simulink model "Examenmodelado_Campoy"  (R2023a)
settings: Solver=VariableStepAuto  StartTime=0.0  StopTime=10.0  RelTol=1e-3
libraries: fl_lib x14, nesl_utility x6, slpidlib x1
settings Model: Creator=marco  LastModifiedBy=marco

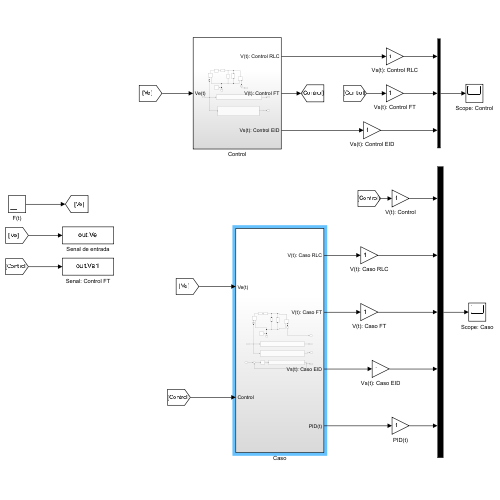
[thumbnail: Simulink's stored preview of the top-level diagram]
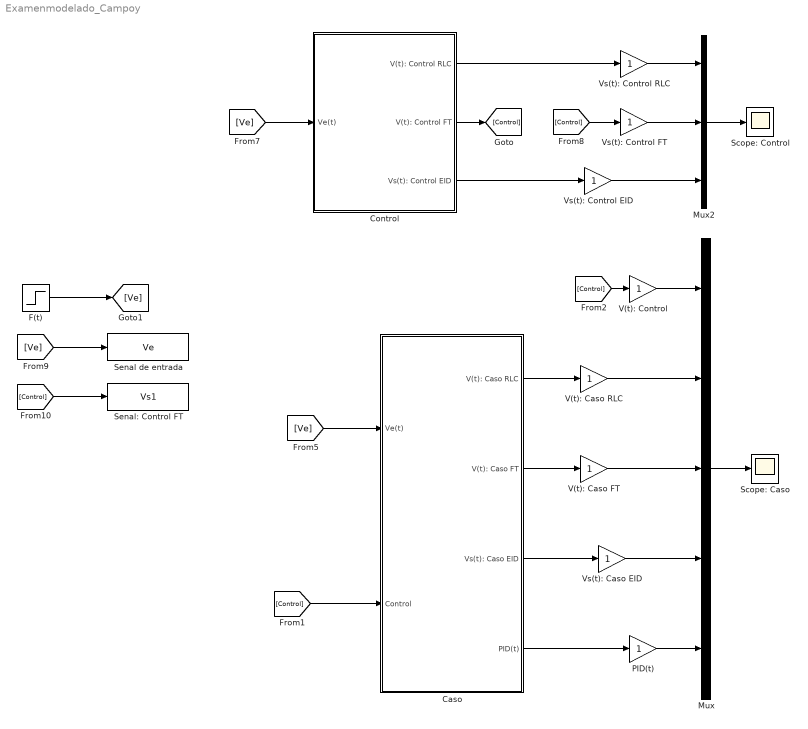
== system Examenmodelado_Campoy ==
  Caso : Subsystem
  Control : Subsystem
  F(t) : Step  SampleTime=0
  Mux : Mux  Inputs=5
  Mux2 : Mux  Inputs=3
  PID(t) : Gain
  Scope: Caso : Scope
  Scope: Control : Scope
  Senal de entrada : ToWorkspace  VariableName=Ve  SampleTime=-1
  Senal: Control FT : ToWorkspace  VariableName=Vs1  SampleTime=-1
  V(t): Caso FT : Gain
  V(t): Caso RLC : Gain
  V(t): Control : Gain
  Vs(t): Caso EID : Gain
  Vs(t): Control EID : Gain
  Vs(t): Control FT : Gain
  Vs(t): Control RLC : Gain
  wires:
  Vs(t): Control EID/1 -> Mux2/3
  V(t): Control/1 -> Mux/1
  Control/2(V(t): Control FT) -> [Control]
  Vs(t): Control RLC/1 -> Mux2/1
  Caso/3(Vs(t): Caso EID) -> Vs(t): Caso EID/1
  [Control] -> Vs(t): Control FT/1
  [Control] -> Senal: Control FT/1
  [Ve] -> Control/1(Ve(t))
  Control/1(V(t): Control RLC) -> Vs(t): Control RLC/1
  Vs(t): Control FT/1 -> Mux2/2
  Mux2/1 -> Scope: Control/1
  Control/3(Vs(t): Control EID) -> Vs(t): Control EID/1
  F(t)/1 -> [Ve]
  Mux/1 -> Scope: Caso/1
  [Ve] -> Senal de entrada/1
  [Control] -> V(t): Control/1
  Caso/2(V(t): Caso FT) -> V(t): Caso FT/1
  Caso/4(PID(t)) -> PID(t)/1
  Vs(t): Caso EID/1 -> Mux/4
  PID(t)/1 -> Mux/5
  [Control] -> Caso/2(Control)
  [Ve] -> Caso/1(Ve(t))
  Caso/1(V(t): Caso RLC) -> V(t): Caso RLC/1
  V(t): Caso RLC/1 -> Mux/2
  V(t): Caso FT/1 -> Mux/3

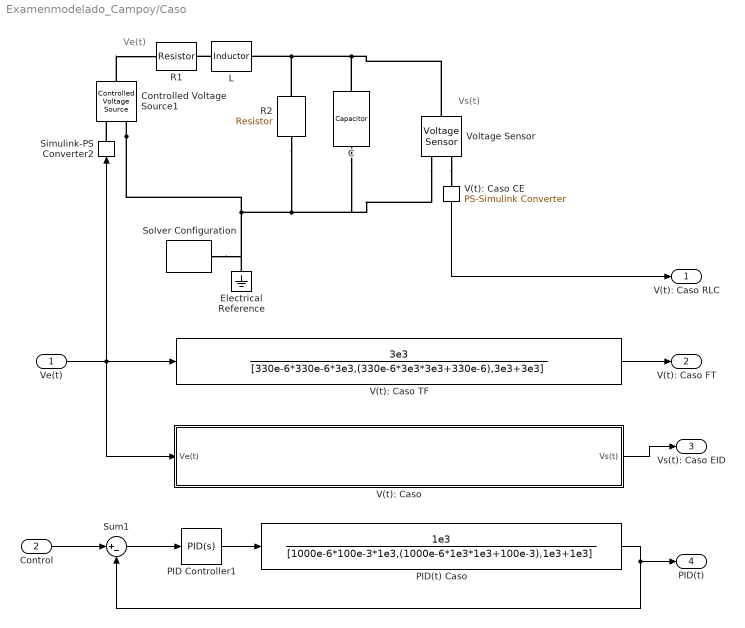
== system Examenmodelado_Campoy/Caso ==
  note: Ve(t)
  note: Vs(t)
  Ve(t) : Inport
  Control : Inport  Port=2
  C : fl_lib/Electrical/Electrical Elements/Capacitor  c=330 uF  r=1e-6 Ohm  g=0 1/Ohm  i_specify=off  i_priority=None  i=0 A  i_nominal_specify=off  i_nominal_unit=A  i_nominal_value=1  v_specify=off  v_priority=None  v=0 V  v_nominal_specify=off  v_nominal_unit=V  v_nominal_value=1  vc_specify=off  vc_priority=High  vc=0 V  vc_nominal_specify=off  vc_nominal_unit=V  vc_nominal_value=1
  Controlled Voltage Source1 : fl_lib/Electrical/Electrical Sources/Controlled Voltage Source
  Electrical Reference : fl_lib/Electrical/Electrical Elements/Electrical Reference
  L : fl_lib/Electrical/Electrical Elements/Inductor  l=330 uH  r=0 Ohm  g=1e-9 1/Ohm  i_specify=off  i_priority=None  i=0 A  i_nominal_specify=off  i_nominal_unit=A  i_nominal_value=1  v_specify=off  v_priority=None  v=0 V  v_nominal_specify=off  v_nominal_unit=V  v_nominal_value=1  i_L_specify=off  i_L_priority=High  i_L=0 A  i_L_nominal_specify=off  i_L_nominal_unit=A  i_L_nominal_value=1
  PID Controller1 : slpidlib/PID Controller  Controller=PID  Form=Parallel  TimeDomain=Continuous-time  UseExternalTs=off  SampleTime=-1  IntegratorMethod=Forward Euler  FilterMethod=Forward Euler  ControllerParametersSource=internal  P=1300.02549518255  I=307059.160027012  UseKiTs=off  D=0.293182881329496  N=7462.72432566653  UseFilter=on  TunerSelectOption=Frequency Response Based  InitialConditionSource=internal  InitialConditionForIntegrator=0  InitialConditionForFilter=0  DifferentiatorICPrevScaledInput=0  ExternalReset=none  TrackingMode=off  Kt=1  LimitOutput=off  SatLimitsSource=internal  UpperSaturationLimit=inf  LowerSaturationLimit=-inf  LinearizeAsGain=on  AntiWindupMode=none  Kb=1  LimitIntegrator=off  UpperIntegratorSaturationLimit=inf  LowerIntegratorSaturationLimit=-inf  POutMin=[]  POutMax=[]  IOutMin=[]  IOutMax=[]  DOutMin=[]  DOutMax=[]  NOutMin=[]  NOutMax=[]  SumOutMin=[]  SumOutMax=[]  SaturationOutMin=[]  SaturationOutMax=[]  PParamMin=[]  PParamMax=[]  IParamMin=[]  IParamMax=[]  DParamMin=[]  DParamMax=[]  NParamMin=[]  NParamMax=[]  KbParamMin=[]  KbParamMax=[]  KtParamMin=[]  KtParamMax=[]  KbOutMin=[]  KbOutMax=[]  KtOutMin=[]  KtOutMax=[]  IntegratorOutMin=[]  IntegratorOutMax=[]  FilterOutMin=[]  FilterOutMax=[]  SumI1OutMin=[]  SumI1OutMax=[]  SumI2OutMin=[]  SumI2OutMax=[]  SumI3OutMin=[]  SumI3OutMax=[]  SumI4OutMin=[]  SumI4OutMax=[]  SumDOutMin=[]  SumDOutMax=[]  DifferentiatorOutMin=[]  DifferentiatorOutMax=[]  FilterDiffOutCoefMin=[]  FilterDiffOutCoefMax=[]  ReciprocalOutMin=[]  ReciprocalOutMax=[]  SumDenOutMin=[]  SumDenOutMax=[]  SumNumOutMin=[]  SumNumOutMax=[]  DivideOutMin=[]  DivideOutMax=[]  UdiffTsProdOutMin=[]  UdiffTsProdOutMax=[]  NTsProdOutMin=[]  NTsProdOutMax=[]  UintegralTsProdOutMin=[]  UintegralTsProdOutMax=[]  UngainTsProdOutMin=[]  UngainTsProdOutMax=[]  ClampingZeroOutDataTypeStr=Inherit: Inherit via back propagation  ClampingZeroOutMin=[]  ClampingZeroOutMax=[]  FilterDenConstantOutDataTypeStr=Inherit: Inherit via back propagation  FilterDenConstantOutMin=[]  FilterDenConstantOutMax=[]  PCopyOutDataTypeStr=Inherit: Inherit via back propagation  PCopyOutMin=[]  PCopyOutMax=[]  NCopyOutDataTypeStr=Inherit: Inherit via back propagation  NCopyOutMin=[]  NCopyOutMax=[]  IntegratorContinuousStateAttributes=''  IntegratorStateMustResolveToSignalObject=off  IntegratorRTWStateStorageClass=Auto  FilterContinuousStateAttributes=''  FilterStateMustResolveToSignalObject=off  FilterRTWStateStorageClass=Auto  ParallelPVariant=InternalParameters  IdealPVariant=Disabled  IVariant=InternalParameters  DVariant=InternalParameters  IntegratorVariant=Continuous  SatVariant=Disabled  AWVariant=Passthrough  PCopyVariant=Disabled  TRVariant=Disabled  FdbkBlocksVariant=Forward  IdealPFdbkVariant=Disabled  SatFdbkVariant=Disabled  DerivativeFilterVariant=ContFilter  NVariant=InternalParameters  NCopyVariant=Disabled  FilterICVariant=InternalICsFilter  IntegratorICVariant=InternalICs  ExternalResetVariant=Disabled  TRSumVariant=Passthrough  SumFdbkVariant=Disabled  SumVariant=Sum_PID  TsampFilterVariant=InternalTs  TsampNgainVariant=Passthrough  TsampIntegralVariant=Disabled_SignalSpec  ExternalSaturationOutDataTypeStr=Inherit: Same as second input
  PID(t) Caso : TransferFcn  Numerator=[1e3]  Denominator=[1000e-6*100e-3*1e3,(1000e-6*1e3*1e3+100e-3),1e3+1e3]
  R1 : fl_lib/Electrical/Electrical Elements/Resistor  R=3 kOhm  i_specify=off  i_priority=None  i=0 A  i_nominal_specify=off  i_nominal_unit=A  i_nominal_value=1  v_specify=off  v_priority=None  v=0 V  v_nominal_specify=off  v_nominal_unit=V  v_nominal_value=1
  R2 : fl_lib/Electrical/Electrical Elements/Resistor  R=3 kOhm  i_specify=off  i_priority=None  i=0 A  i_nominal_specify=off  i_nominal_unit=A  i_nominal_value=1  v_specify=off  v_priority=None  v=0 V  v_nominal_specify=off  v_nominal_unit=V  v_nominal_value=1
  Simulink-PS Converter2 : nesl_utility/Simulink-PS Converter  PhysicalDomain=network_engine_domain  SubClassName=ps_input  LeftPortType=input  RightPortType=output  PseudoPeriodic=off  Frequencies=[]  NoiseDistribution=none  NoiseParameters=[]  Unit=1  AffineConversion=off  FilteringAndDerivatives=provide  SimscapeFilterOrder=1  InputFilterTimeConstant=0.001  UdotUserProvided=0
  Solver Configuration : nesl_utility/Solver Configuration  PhysicalDomain=network_engine_domain  SubClassName=solver  LeftPortType=input  RightPortType=generic  Tones=[]  Harmonics=[]  SimulateNoise=off  Profile=off  UseLocalSampling=off  EnableSwitchedLinearOptims=on  FrequencyDomain=off  UseCCode=off  RelTol=0.001  AbsTol=1e-06  MinStep=1e-09  ToWorkspace=off  RevertToSquareIcSolve=off  NumHomotopyIterations=100  PhasorMode=off  PhasorModeNumHarmonics=1  ConsistencySolver=NEWTON_FTOL  IndexReductionMethod=DerivativeReplacement  DoDC=off  ResidualTolerance=1e-09  ConsistencyTolSource=GLOBAL  ConsistencyAbsTol=0.001  ConsistencyRelTol=0.001  ConsistencyTolFactor=0.001  UseLocalSolver=off  LocalSolverChoice=NE_BACKWARD_EULER_ADVANCER  ResolveIndetEquations=on  FunctionEvalNumThread=1  LocalSolverSampleTime=0.001  DoFixedCost=off  MaxNonlinIter=3  MaxModeIter=2  ComputeImpulses=off  ImpulseIterations=2  LinearAlgebra=auto  LinearAlgebraNumThread=0  EquationFormulation=NE_TIME_EF  DelaysMemoryBudget=1024  AutomaticFiltering=on  FilteringTimeConstant=0.001  PartitionStorageMethod=AS_NEEDED  PartitionMemoryBudget=1024  PartitionMethod=ROBUST
  Sum1 : Sum  Inputs=|+-
  V(t): Caso : Subsystem
  V(t): Caso CE : nesl_utility/PS-Simulink Converter  PhysicalDomain=network_engine_domain  SubClassName=ps_output  LeftPortType=input  RightPortType=output  PseudoPeriodic=off  Frequencies=[]  VectorFormat=1-D array  Unit=inherit  AffineConversion=off
  V(t): Caso TF : TransferFcn  Numerator=[3e3]  Denominator=[330e-6*330e-6*3e3,(330e-6*3e3*3e3+330e-6),3e3+3e3]
  Voltage Sensor : fl_lib/Electrical/Electrical Sensors/Voltage Sensor
  V(t): Caso RLC : Outport
  V(t): Caso FT : Outport  Port=2
  Vs(t): Caso EID : Outport  Port=3
  PID(t) : Outport  Port=4
  wires:
  Sum1/1 -> PID Controller1/1
  PID(t) Caso/1 -> PID(t)/1, Sum1/2
  Control/1 -> Sum1/1
  PID Controller1/1 -> PID(t) Caso/1
  V(t): Caso TF/1 -> V(t): Caso FT/1
  V(t): Caso CE/1 -> V(t): Caso RLC/1
  Ve(t)/1 -> V(t): Caso/1(Ve(t)), V(t): Caso TF/1, Simulink-PS Converter2/1
  V(t): Caso/1(Vs(t)) -> Vs(t): Caso EID/1
  connections:
  Controlled Voltage Source1/RConn2 -- Voltage Sensor/RConn2 -- C/RConn1 -- R2/RConn1 -- Electrical Reference/LConn1 -- Solver Configuration/RConn1
  L/LConn1 -- R1/RConn1
  Voltage Sensor/LConn1 -- L/RConn1 -- R2/LConn1 -- C/LConn1
  Simulink-PS Converter2/RConn1 -- Controlled Voltage Source1/RConn1
  Voltage Sensor/RConn1 -- V(t): Caso CE/LConn1
  Controlled Voltage Source1/LConn1 -- R1/LConn1

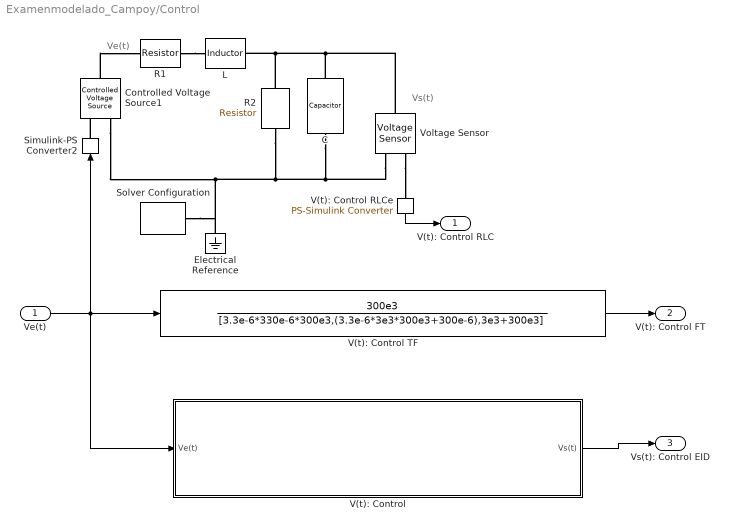
== system Examenmodelado_Campoy/Control ==
  note: Ve(t)
  note: Vs(t)
  Ve(t) : Inport
  C : fl_lib/Electrical/Electrical Elements/Capacitor  c=3.3 uF  r=1e-6 Ohm  g=0 1/Ohm  i_specify=off  i_priority=None  i=0 A  i_nominal_specify=off  i_nominal_unit=A  i_nominal_value=1  v_specify=off  v_priority=None  v=0 V  v_nominal_specify=off  v_nominal_unit=V  v_nominal_value=1  vc_specify=off  vc_priority=High  vc=0 V  vc_nominal_specify=off  vc_nominal_unit=V  vc_nominal_value=1
  Controlled Voltage Source1 : fl_lib/Electrical/Electrical Sources/Controlled Voltage Source
  Electrical Reference : fl_lib/Electrical/Electrical Elements/Electrical Reference
  L : fl_lib/Electrical/Electrical Elements/Inductor  l=330 uH  r=0 Ohm  g=1e-9 1/Ohm  i_specify=off  i_priority=None  i=0 A  i_nominal_specify=off  i_nominal_unit=A  i_nominal_value=1  v_specify=off  v_priority=None  v=0 V  v_nominal_specify=off  v_nominal_unit=V  v_nominal_value=1  i_L_specify=off  i_L_priority=High  i_L=0 A  i_L_nominal_specify=off  i_L_nominal_unit=A  i_L_nominal_value=1
  R1 : fl_lib/Electrical/Electrical Elements/Resistor  R=3 kOhm  i_specify=off  i_priority=None  i=0 A  i_nominal_specify=off  i_nominal_unit=A  i_nominal_value=1  v_specify=off  v_priority=None  v=0 V  v_nominal_specify=off  v_nominal_unit=V  v_nominal_value=1
  R2 : fl_lib/Electrical/Electrical Elements/Resistor  R=300 kOhm  i_specify=off  i_priority=None  i=0 A  i_nominal_specify=off  i_nominal_unit=A  i_nominal_value=1  v_specify=off  v_priority=None  v=0 V  v_nominal_specify=off  v_nominal_unit=V  v_nominal_value=1
  Simulink-PS Converter2 : nesl_utility/Simulink-PS Converter  PhysicalDomain=network_engine_domain  SubClassName=ps_input  LeftPortType=input  RightPortType=output  PseudoPeriodic=off  Frequencies=[]  NoiseDistribution=none  NoiseParameters=[]  Unit=1  AffineConversion=off  FilteringAndDerivatives=provide  SimscapeFilterOrder=1  InputFilterTimeConstant=0.001  UdotUserProvided=0
  Solver Configuration : nesl_utility/Solver Configuration  PhysicalDomain=network_engine_domain  SubClassName=solver  LeftPortType=input  RightPortType=generic  Tones=[]  Harmonics=[]  SimulateNoise=off  Profile=off  UseLocalSampling=off  EnableSwitchedLinearOptims=on  FrequencyDomain=off  UseCCode=off  RelTol=0.001  AbsTol=1e-06  MinStep=1e-09  ToWorkspace=off  RevertToSquareIcSolve=off  NumHomotopyIterations=100  PhasorMode=off  PhasorModeNumHarmonics=1  ConsistencySolver=NEWTON_FTOL  IndexReductionMethod=DerivativeReplacement  DoDC=off  ResidualTolerance=1e-09  ConsistencyTolSource=GLOBAL  ConsistencyAbsTol=0.001  ConsistencyRelTol=0.001  ConsistencyTolFactor=0.001  UseLocalSolver=off  LocalSolverChoice=NE_BACKWARD_EULER_ADVANCER  ResolveIndetEquations=on  FunctionEvalNumThread=1  LocalSolverSampleTime=0.001  DoFixedCost=off  MaxNonlinIter=3  MaxModeIter=2  ComputeImpulses=off  ImpulseIterations=2  LinearAlgebra=auto  LinearAlgebraNumThread=0  EquationFormulation=NE_TIME_EF  DelaysMemoryBudget=1024  AutomaticFiltering=on  FilteringTimeConstant=0.001  PartitionStorageMethod=AS_NEEDED  PartitionMemoryBudget=1024  PartitionMethod=ROBUST
  V(t): Control : Subsystem
  V(t): Control RLCe : nesl_utility/PS-Simulink Converter  PhysicalDomain=network_engine_domain  SubClassName=ps_output  LeftPortType=input  RightPortType=output  PseudoPeriodic=off  Frequencies=[]  VectorFormat=1-D array  Unit=inherit  AffineConversion=off
  V(t): Control TF : TransferFcn  Numerator=[300e3]  Denominator=[3.3e-6*330e-6*300e3,(3.3e-6*3e3*300e3+300e-6),3e3+300e3]
  Voltage Sensor : fl_lib/Electrical/Electrical Sensors/Voltage Sensor
  V(t): Control RLC : Outport
  V(t): Control FT : Outport  Port=2
  Vs(t): Control EID : Outport  Port=3
  wires:
  Ve(t)/1 -> V(t): Control/1(Ve(t)), V(t): Control TF/1, Simulink-PS Converter2/1
  V(t): Control RLCe/1 -> V(t): Control RLC/1
  V(t): Control TF/1 -> V(t): Control FT/1
  V(t): Control/1(Vs(t)) -> Vs(t): Control EID/1
  connections:
  Voltage Sensor/RConn1 -- V(t): Control RLCe/LConn1
  Simulink-PS Converter2/RConn1 -- Controlled Voltage Source1/RConn1
  Voltage Sensor/LConn1 -- C/LConn1 -- R2/LConn1 -- L/RConn1
  Voltage Sensor/RConn2 -- C/RConn1 -- R2/RConn1 -- Electrical Reference/LConn1 -- Solver Configuration/RConn1 -- Controlled Voltage Source1/RConn2
  Controlled Voltage Source1/LConn1 -- R1/LConn1
  R1/RConn1 -- L/LConn1

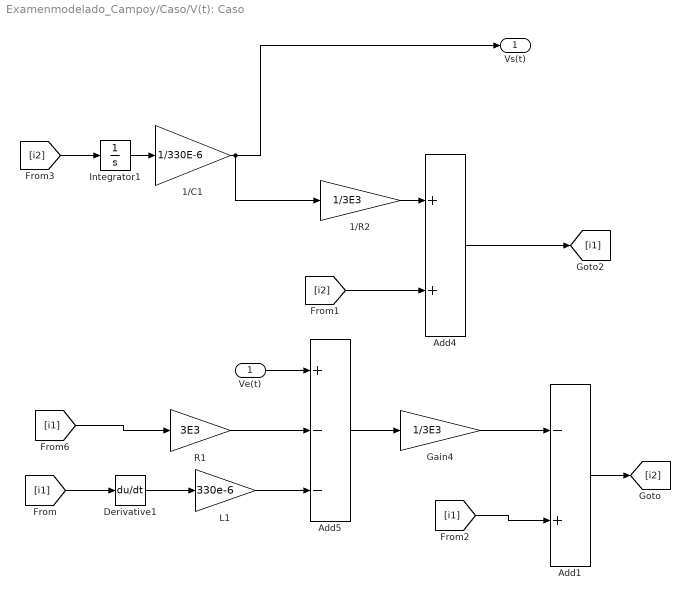
== system Examenmodelado_Campoy/Caso/V(t): Caso ==
  Ve(t) : Inport
  1/C1 : Gain  Gain=1/330E-6
  1/R2 : Gain  Gain=1/3E3
  Add1 : Sum  Inputs=-+
  Add4 : Sum
  Add5 : Sum  Inputs=+--
  Derivative1 : Derivative
  Gain4 : Gain  Gain=1/3E3
  Integrator1 : Integrator
  L1 : Gain  Gain=330e-6
  R1 : Gain  Gain=3E3
  Vs(t) : Outport
  wires:
  Integrator1/1 -> 1/C1/1
  [i2] -> Integrator1/1
  1/C1/1 -> 1/R2/1, Vs(t)/1
  1/R2/1 -> Add4/1
  [i1] -> Derivative1/1
  Derivative1/1 -> L1/1
  L1/1 -> Add5/3
  R1/1 -> Add5/2
  Ve(t)/1 -> Add5/1
  Add5/1 -> Gain4/1
  [i1] -> R1/1
  Add4/1 -> [i1]
  [i2] -> Add4/2
  Gain4/1 -> Add1/1
  [i1] -> Add1/2
  Add1/1 -> [i2]

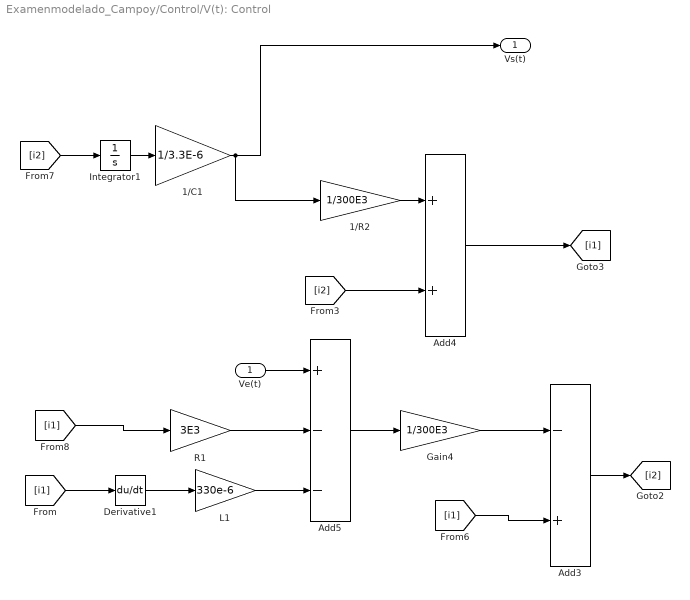
== system Examenmodelado_Campoy/Control/V(t): Control ==
  Ve(t) : Inport
  1/C1 : Gain  Gain=1/3.3E-6
  1/R2 : Gain  Gain=1/300E3
  Add3 : Sum  Inputs=-+
  Add4 : Sum
  Add5 : Sum  Inputs=+--
  Derivative1 : Derivative
  Gain4 : Gain  Gain=1/300E3
  Integrator1 : Integrator
  L1 : Gain  Gain=330e-6
  R1 : Gain  Gain=3E3
  Vs(t) : Outport
  wires:
  1/C1/1 -> 1/R2/1, Vs(t)/1
  [i1] -> Derivative1/1
  [i2] -> Integrator1/1
  Add3/1 -> [i2]
  [i1] -> Add3/2
  Gain4/1 -> Add3/1
  Add5/1 -> Gain4/1
  1/R2/1 -> Add4/1
  [i2] -> Add4/2
  Add4/1 -> [i1]
  Derivative1/1 -> L1/1
  Integrator1/1 -> 1/C1/1
  Ve(t)/1 -> Add5/1
  [i1] -> R1/1
  R1/1 -> Add5/2
  L1/1 -> Add5/3
